simulink model "buffer_silo"  (Simulink 9.2)
settings: Solver=VariableStepAuto  StartTime=0.0  StopTime=500  RelTol=1e-3
values from neighbouring files (symbols this model uses):
  beta = 46.5    [main.m]
  comp = 1    [main.m]
  H_step = H_star_out.Data / MT_step / Kp    [main.m]
  Kc = 2    [main.m]
  Kd = 8    [main.m]
  Kd1 = 15    [main.m]
  Kd2 = 14    [main.m]
  Kep_1 = 2    [main.m]
  Kep_2 = 2    [main.m]
  Kh = 1.4    [main.m]
  Ki1 = 0.065    [main.m]
  Ki2 = 0.1    [main.m]
  Km = 0.185    [main.m]
  Kp = 1/beta    (= 0.0215053763441)    [main.m]
  Kp1 = 2.2    [main.m]
  Kp2 = 7    [main.m]
  Mo_step = Mo_star_out.Data / MT_step    [main.m]
  MT_amp = 0    [main.m]
  MT_freq = 0.08    [main.m]
  MT_step = 1    [main.m]
  noiseamp = 0.1    [main.m]
  tauc = 25    [main.m]
  taud = 25    [main.m]
  taum = 0.5    [main.m]
  taup = rho * AT / beta    (= 60.2150537634)    [main.m]
  tdelay = 1    [main.m]
libraries: simulink x2
settings Model: Creator=andreinicusan  LastModifiedBy=andreinicusan
settings DataIOCC: LimitDataPoints=off  SaveFormat=Dataset  SignalLoggingSaveFormat=Dataset
settings OptimizationCC: LifeSpan=auto
settings DebuggingCC: UnderspecifiedInitializationDetection=Simplified  MergeDetectMultiDrivingBlocksExec=error  FcnCallInpInsideContextMsg=error  StateNameClashWarn=none  SFUnexpectedBacktrackingDiag=error  SFNoUnconditionalDefaultTransitionDiag=error  SFExecutionAtInitializationDiag=warning
settings HardwareCC: ProdBitPerPointer=64  ProdBitPerSizeT=64  ProdBitPerPtrDiffT=64  ProdLargestAtomicFloat=Float  ProdIntDivRoundTo=Zero  ProdEndianess=LittleEndian  ProdWordSize=64  ProdHWDeviceType=Intel->x86-64 (Windows64)
settings ModelReferenceCC: PropagateSignalLabelsOutOfModel=on
settings SFSimCC: SimUseLocalCustomCode=on
settings RTWCC: RTWUseLocalCustomCode=on
settings CodeAppCC: StateflowObjectComments=off
settings GRTTargetCC: TargetLangStandard=C99 (ISO)  GeneratePreprocessorConditionals=Use local settings  CombineOutputUpdateFcns=on  GRTInterface=off
settings ConfigComp: CovMetricSettings=dwe  CovHtmlReporting=off  CovSaveCumulativeToWorkspaceVar=off  CovSaveSingleToWorkspaceVar=off  CovExternalEMLEnable=on

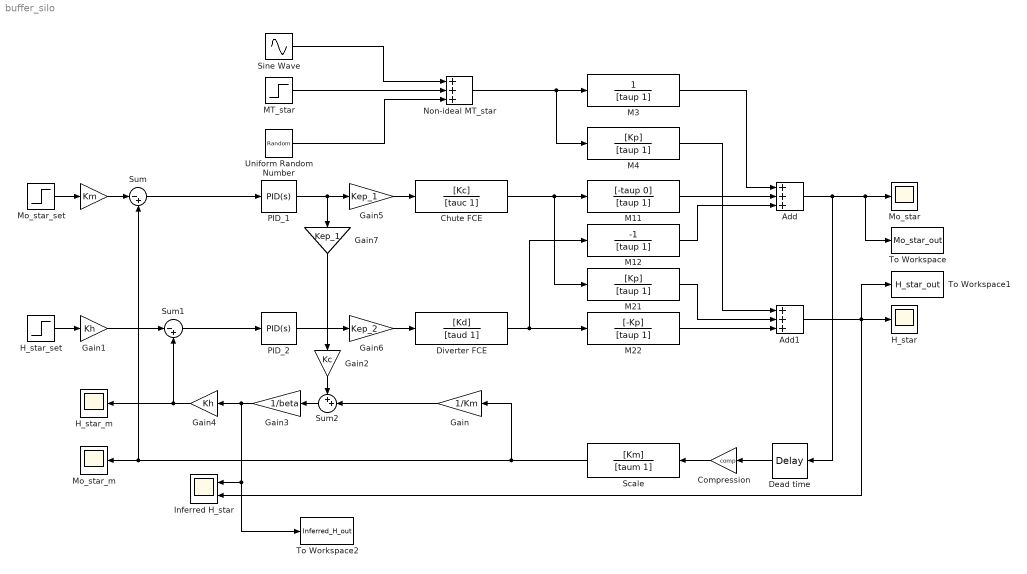
== system buffer_silo ==
  " " : Gain  Gain=Km
  Add : Sum  Inputs=+++
  Add1 : Sum  Inputs=+++
  Chute FCE : TransferFcn  Numerator=[Kc]  Denominator=[tauc 1]
  Compression : Gain  Gain=comp
  Dead time : TransportDelay  DelayTime=tdelay
  Diverter FCE : TransferFcn  Numerator=[Kd]  Denominator=[taud 1]
  Gain : Gain  Gain=1/Km
  Gain1 : Gain  Gain=Kh
  Gain2 : Gain  Gain=Kc
  Gain3 : Gain  Gain=1/beta
  Gain4 : Gain  Gain=Kh
  Gain5 : Gain  Gain=Kep_1
  Gain6 : Gain  Gain=Kep_2
  Gain7 : Gain  Gain=Kep_1
  H_star : Scope
  H_star_m : Scope
  H_star_set : Step  After=H_step  SampleTime=0
  Inferred H_star : Scope  NumInputPorts=2
  M11 : TransferFcn  Numerator=[-taup 0]  Denominator=[taup 1]
  M12 : TransferFcn  Numerator=[-1]  Denominator=[taup 1]
  M21 : TransferFcn  Numerator=[Kp]  Denominator=[taup 1]
  M22 : TransferFcn  Numerator=[-Kp]  Denominator=[taup 1]
  M3 : TransferFcn  Denominator=[taup 1]
  M4 : TransferFcn  Numerator=[Kp]  Denominator=[taup 1]
  MT_star : Step  After=MT_step  SampleTime=0
  Mo_star : Scope
  Mo_star_m : Scope
  Mo_star_set : Step  After=Mo_step  SampleTime=0
  Non-ideal MT_star : Sum  Inputs=+++
  PID_1 : simulink/Continuous/PID Controller  Controller=PID  Form=Parallel  TimeDomain=Continuous-time  SampleTime=-1  IntegratorMethod=Forward Euler  FilterMethod=Forward Euler  ControllerParametersSource=internal  P=Kp1  I=Ki1  D=Kd1  UseFilter=on  N=100  TunerSelectOption=Transfer Function Based (PID Tuner App)  InitialConditionSource=internal  InitialConditionForIntegrator=0  InitialConditionForFilter=0  DifferentiatorICPrevScaledInput=0  ExternalReset=none  TrackingMode=off  Kt=1  LimitOutput=off  UpperSaturationLimit=inf  LowerSaturationLimit=-inf  LinearizeAsGain=on  AntiWindupMode=none  Kb=1  POutMin=[]  POutMax=[]  IOutMin=[]  IOutMax=[]  DOutMin=[]  DOutMax=[]  NOutMin=[]  NOutMax=[]  SumOutMin=[]  SumOutMax=[]  SaturationOutMin=[]  SaturationOutMax=[]  PParamMin=[]  PParamMax=[]  IParamMin=[]  IParamMax=[]  DParamMin=[]  DParamMax=[]  NParamMin=[]  NParamMax=[]  KbParamMin=[]  KbParamMax=[]  KtParamMin=[]  KtParamMax=[]  KbOutMin=[]  KbOutMax=[]  KtOutMin=[]  KtOutMax=[]  IntegratorOutMin=[]  IntegratorOutMax=[]  FilterOutMin=[]  FilterOutMax=[]  SumI1OutMin=[]  SumI1OutMax=[]  SumI2OutMin=[]  SumI2OutMax=[]  SumI3OutMin=[]  SumI3OutMax=[]  SumI4OutMin=[]  SumI4OutMax=[]  SumDOutMin=[]  SumDOutMax=[]  DifferentiatorOutMin=[]  DifferentiatorOutMax=[]  FilterDiffOutCoefMin=[]  FilterDiffOutCoefMax=[]  ReciprocalOutMin=[]  ReciprocalOutMax=[]  SumDenOutMin=[]  SumDenOutMax=[]  SumNumOutMin=[]  SumNumOutMax=[]  DivideOutMin=[]  DivideOutMax=[]  IntegratorContinuousStateAttributes=''  IntegratorStateMustResolveToSignalObject=off  IntegratorRTWStateStorageClass=Auto  FilterContinuousStateAttributes=''  FilterStateMustResolveToSignalObject=off  FilterRTWStateStorageClass=Auto  ParallelPVariant=InternalParameters  IdealPVariant=Disabled  IVariant=InternalParameters  DVariant=InternalParameters  IntegratorVariant=Continuous  SatVariant=Disabled  AWVariant=Passthrough  PCopyVariant=Disabled  TRVariant=Disabled  FdbkBlocksVariant=Forward  IdealPFdbkVariant=Disabled  SatFdbkVariant=Disabled  DerivativeFilterVariant=ContFilter  NVariant=InternalParameters  NCopyVariant=Disabled  FilterICVariant=InternalICsFilter  IntegratorICVariant=InternalICs  ExternalResetVariant=Disabled  TRSumVariant=Passthrough  SumFdbkVariant=Disabled  SumVariant=Sum_PID
  PID_2 : simulink/Continuous/PID Controller  Controller=PID  Form=Parallel  TimeDomain=Continuous-time  SampleTime=-1  IntegratorMethod=Forward Euler  FilterMethod=Forward Euler  ControllerParametersSource=internal  P=Kp2  I=Ki2  D=Kd2  UseFilter=on  N=100  TunerSelectOption=Transfer Function Based (PID Tuner App)  InitialConditionSource=internal  InitialConditionForIntegrator=0  InitialConditionForFilter=0  DifferentiatorICPrevScaledInput=0  ExternalReset=none  TrackingMode=off  Kt=1  LimitOutput=off  UpperSaturationLimit=inf  LowerSaturationLimit=-inf  LinearizeAsGain=on  AntiWindupMode=none  Kb=1  POutMin=[]  POutMax=[]  IOutMin=[]  IOutMax=[]  DOutMin=[]  DOutMax=[]  NOutMin=[]  NOutMax=[]  SumOutMin=[]  SumOutMax=[]  SaturationOutMin=[]  SaturationOutMax=[]  PParamMin=[]  PParamMax=[]  IParamMin=[]  IParamMax=[]  DParamMin=[]  DParamMax=[]  NParamMin=[]  NParamMax=[]  KbParamMin=[]  KbParamMax=[]  KtParamMin=[]  KtParamMax=[]  KbOutMin=[]  KbOutMax=[]  KtOutMin=[]  KtOutMax=[]  IntegratorOutMin=[]  IntegratorOutMax=[]  FilterOutMin=[]  FilterOutMax=[]  SumI1OutMin=[]  SumI1OutMax=[]  SumI2OutMin=[]  SumI2OutMax=[]  SumI3OutMin=[]  SumI3OutMax=[]  SumI4OutMin=[]  SumI4OutMax=[]  SumDOutMin=[]  SumDOutMax=[]  DifferentiatorOutMin=[]  DifferentiatorOutMax=[]  FilterDiffOutCoefMin=[]  FilterDiffOutCoefMax=[]  ReciprocalOutMin=[]  ReciprocalOutMax=[]  SumDenOutMin=[]  SumDenOutMax=[]  SumNumOutMin=[]  SumNumOutMax=[]  DivideOutMin=[]  DivideOutMax=[]  IntegratorContinuousStateAttributes=''  IntegratorStateMustResolveToSignalObject=off  IntegratorRTWStateStorageClass=Auto  FilterContinuousStateAttributes=''  FilterStateMustResolveToSignalObject=off  FilterRTWStateStorageClass=Auto  ParallelPVariant=InternalParameters  IdealPVariant=Disabled  IVariant=InternalParameters  DVariant=InternalParameters  IntegratorVariant=Continuous  SatVariant=Disabled  AWVariant=Passthrough  PCopyVariant=Disabled  TRVariant=Disabled  FdbkBlocksVariant=Forward  IdealPFdbkVariant=Disabled  SatFdbkVariant=Disabled  DerivativeFilterVariant=ContFilter  NVariant=InternalParameters  NCopyVariant=Disabled  FilterICVariant=InternalICsFilter  IntegratorICVariant=InternalICs  ExternalResetVariant=Disabled  TRSumVariant=Passthrough  SumFdbkVariant=Disabled  SumVariant=Sum_PID
  Scale : TransferFcn  Numerator=[Km]  Denominator=[taum 1]
  Sine Wave : Sin  Amplitude=MT_amp  Frequency=MT_freq  SampleTime=0
  Sum : Sum  Inputs=|-+
  Sum1 : Sum  Inputs=|-+
  Sum2 : Sum  Inputs=++|
  To Workspace : ToWorkspace  VariableName=Mo_star_out  SaveFormat=Timeseries  SampleTime=-1
  To Workspace1 : ToWorkspace  VariableName=H_star_out  SaveFormat=Timeseries  SampleTime=-1
  To Workspace2 : ToWorkspace  VariableName=Inferred_H_out  SaveFormat=Timeseries  SampleTime=-1
  Uniform Random Number : UniformRandomNumber  Minimum=-noiseamp  Maximum=noiseamp  SampleTime=0.1
  wires:
  Mo_star_set/1 -> " "/1
  H_star_set/1 -> Gain1/1
  " "/1 -> Sum/1
  Sum/1 -> PID_1/1
  PID_1/1 -> Gain7/1, Gain5/1
  PID_2/1 -> Gain6/1
  Chute FCE/1 -> M21/1, M11/1
  Diverter FCE/1 -> M12/1, M22/1
  M11/1 -> Add/2
  M12/1 -> Add/3
  M22/1 -> Add1/3
  M21/1 -> Add1/2
  Non-ideal MT_star/1 -> M4/1, M3/1
  M3/1 -> Add/1
  M4/1 -> Add1/1
  Add/1 -> Dead time/1, To Workspace/1, Mo_star/1
  Add1/1 -> To Workspace1/1, H_star/1, Inferred H_star/2
  Scale/1 -> Gain/1, Mo_star_m/1, Sum/2
  Gain2/1 -> Sum2/1
  Gain/1 -> Sum2/2
  Sum2/1 -> Gain3/1
  Gain4/1 -> Sum1/2, H_star_m/1
  Gain1/1 -> Sum1/1
  Sum1/1 -> PID_2/1
  Gain3/1 -> Gain4/1, To Workspace2/1, Inferred H_star/1
  Sine Wave/1 -> Non-ideal MT_star/1
  MT_star/1 -> Non-ideal MT_star/2
  Uniform Random Number/1 -> Non-ideal MT_star/3
  Gain5/1 -> Chute FCE/1
  Gain6/1 -> Diverter FCE/1
  Gain7/1 -> Gain2/1
  Dead time/1 -> Compression/1
  Compression/1 -> Scale/1
